simulink model "LAB_02_26_SEPT_SIM_SMD"  (R2022b)
settings: Solver=VariableStepAuto  StartTime=0.0  StopTime=10.0  RelTol=1e-3
values from neighbouring files (symbols this model uses):
  b = [cos(eps), sin(eps)]    [LAB_01_19_SEPT.m]    (also in LAB_02_26_SEPT_MAT_SMD.m = 5)
  k = 6    [LAB_02_26_SEPT_MAT_SMD.m]
  m = 2    [LAB_02_26_SEPT_MAT_SMD.m]
  omega = 0.5    [LAB_02_26_SEPT_MAT_SMD.m]
  v0 = [3.021; 24.139; 10.964]    [LAB_02_26_SEPT_MAT_2BODYDYN.m]    (also in LAB_02_26_SEPT_MAT_SMD.m = 0)
  x0 = 1    [LAB_02_26_SEPT_MAT_SMD.m]
settings Model: Creator=maria  LastModifiedBy=maria

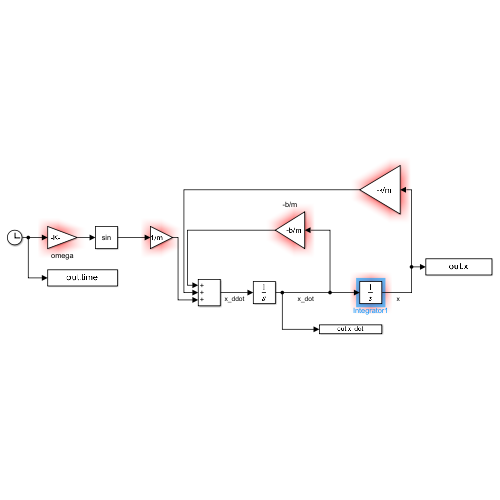
[thumbnail: Simulink's stored preview of the top-level diagram]
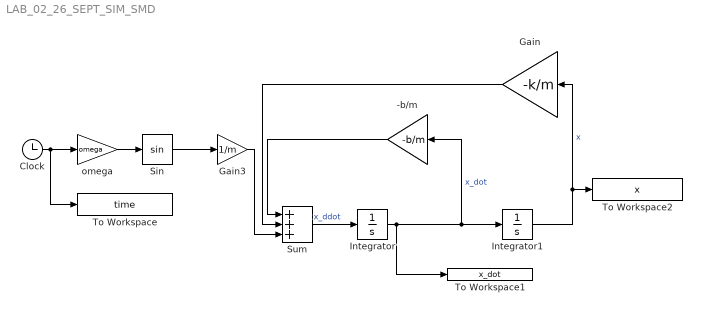
== system LAB_02_26_SEPT_SIM_SMD ==
  -b/m : Gain  Gain=-b/m
  Clock : Clock
  Gain : Gain  Gain=-k/m
  Gain3 : Gain  Gain=1/m
  Integrator : Integrator  InitialCondition=v0
  Integrator1 : Integrator  InitialCondition=x0
  Sin : Trigonometry
  Sum : Sum  Inputs=+++
  To Workspace : ToWorkspace  VariableName=time  SaveFormat=Timeseries  SampleTime=-1
  To Workspace1 : ToWorkspace  VariableName=x_dot  SaveFormat=Timeseries  SampleTime=-1
  To Workspace2 : ToWorkspace  VariableName=x  SaveFormat=Timeseries  SampleTime=-1
  omega : Gain  Gain=omega
  wires:
  Integrator/1 -> To Workspace1/1, -b/m/1, Integrator1/1  "x_dot"
  Integrator1/1 -> To Workspace2/1, Gain/1  "x"
  Sum/1 -> Integrator/1  "x_ddot"
  Clock/1 -> To Workspace/1, omega/1
  omega/1 -> Sin/1
  Sin/1 -> Gain3/1
  Gain3/1 -> Sum/3
  -b/m/1 -> Sum/1
  Gain/1 -> Sum/2
